simulink model "model_2_type"  (R2022b)
settings: Solver=VariableStepAuto  StartTime=0.0  StopTime=2500  MaxStep=1e-3  RelTol=1e-3
undefined symbols (not defined in the file or in its folder): a0, a1, b0, gamma_1, gamma_2, k0, k_M_1, k_M_2
settings Model: Creator=deniskirbaba  LastModifiedBy=R1303-We2-1-Stud
settings OptimizationCC: ReuseModelBlockBuffer=on

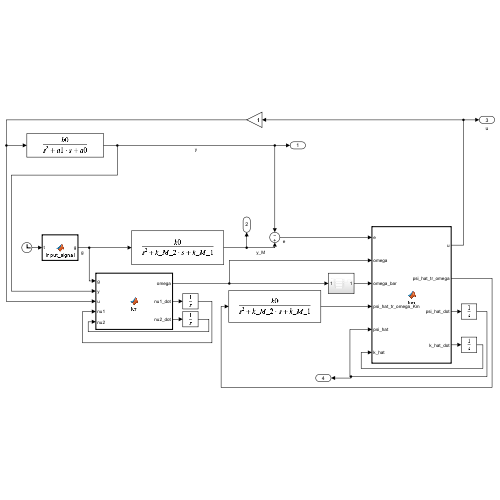
[thumbnail: Simulink's stored preview of the top-level diagram]
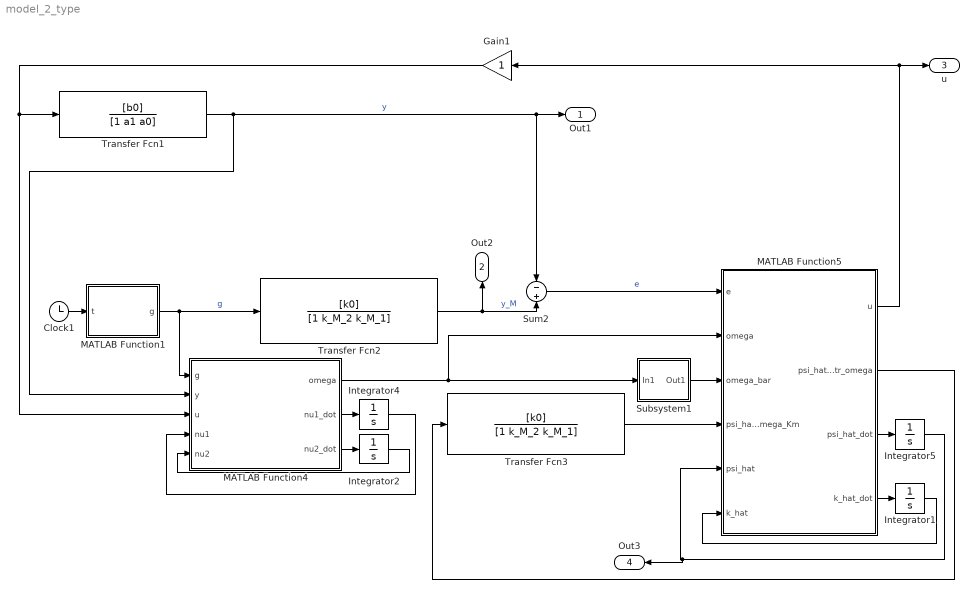
== system model_2_type ==
  Clock1 : Clock
  Gain1 : Gain
  Integrator1 : Integrator
  Integrator2 : Integrator
  Integrator4 : Integrator
  Integrator5 : Integrator  InitialCondition=[0;0;0;0]
  MATLAB Function1 : MATLAB Function  TreatAsAtomicUnit=on
  MATLAB Function4 : MATLAB Function  TreatAsAtomicUnit=on
  MATLAB Function5 : MATLAB Function  TreatAsAtomicUnit=on
  Subsystem1 : Subsystem
  Sum2 : Sum  Inputs=-+
  Transfer Fcn1 : TransferFcn  Numerator=[b0]  Denominator=[1 a1 a0]
  Transfer Fcn2 : TransferFcn  Numerator=[k0]  Denominator=[1 k_M_2 k_M_1]
  Transfer Fcn3 : TransferFcn  Numerator=[k0]  Denominator=[1 k_M_2 k_M_1]
  Out1 : Outport
  Out2 : Outport  Port=2
  u : Outport  Port=3
  Out3 : Outport  Port=4
  wires:
  MATLAB Function4/2(nu1_dot) -> Integrator4/1
  MATLAB Function1/1(g) -> MATLAB Function4/1(g), Transfer Fcn2/1  "g"
  Transfer Fcn2/1 -> Out2/1, Sum2/2  "y_M"
  MATLAB Function5/2(psi_hat_tr_omega) -> Transfer Fcn3/1
  Transfer Fcn3/1 -> MATLAB Function5/4(psi_hat_tr_omega_Km)
  MATLAB Function4/1(omega) -> Subsystem1/1(In1), MATLAB Function5/2(omega)
  Gain1/1 -> MATLAB Function4/3(u), Transfer Fcn1/1
  Clock1/1 -> MATLAB Function1/1(t)
  Subsystem1/1(Out1) -> MATLAB Function5/3(omega_bar)
  Integrator2/1 -> MATLAB Function4/5(nu2)
  Transfer Fcn1/1 -> Out1/1, Sum2/1, MATLAB Function4/2(y)  "y"
  MATLAB Function5/3(psi_hat_dot) -> Integrator5/1
  Integrator4/1 -> MATLAB Function4/4(nu1)
  MATLAB Function4/3(nu2_dot) -> Integrator2/1
  Sum2/1 -> MATLAB Function5/1(e)  "e"
  Integrator5/1 -> Out3/1, MATLAB Function5/5(psi_hat)
  MATLAB Function5/1(u) -> u/1, Gain1/1
  MATLAB Function5/4(k_hat_dot) -> Integrator1/1
  Integrator1/1 -> MATLAB Function5/6(k_hat)

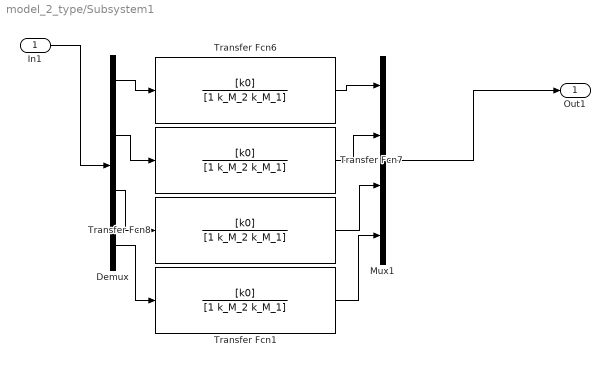
== system model_2_type/Subsystem1 ==
  In1 : Inport
  Demux : Demux
  Mux1 : Mux
  Transfer Fcn{1,6..8} (4 alike) : TransferFcn  Numerator=[k0]  Denominator=[1 k_M_2 k_M_1]
  Out1 : Outport
  wires:
  Transfer Fcn6/1 -> Mux1/1
  Demux/1 -> Transfer Fcn6/1
  Demux/3 -> Transfer Fcn8/1
  Demux/2 -> Transfer Fcn7/1
  Transfer Fcn7/1 -> Mux1/2
  In1/1 -> Demux/1
  Mux1/1 -> Out1/1
  Transfer Fcn8/1 -> Mux1/3
  Demux/4 -> Transfer Fcn1/1
  Transfer Fcn1/1 -> Mux1/4

== matlab function model_2_type/MATLAB Function1 ==
  data: t input; g output
function g = input_signal(t)
    g = sin(t);%7*sign(cos(0.9*t));
end

== matlab function model_2_type/MATLAB Function4 ==
  data: g input; y input; u input; nu1 input; nu2 input; omega output; nu1_dot output; nu2_dot output; k0 parameter
function [omega, nu1_dot, nu2_dot] = fcn(g, y, u, nu1, nu2, k0)
    lambda =-k0;
    
    nu1_dot = lambda*nu1 + u;
    nu2_dot = lambda*nu2 + y;

    omega = [nu1,nu2,y,g]';
end

== matlab function model_2_type/MATLAB Function5 ==
  data: e input; omega input; omega_bar input; psi_hat_tr_omega_Km input; psi_hat input; k_hat input; u output; psi_hat_tr_omega output; psi_hat_dot output; gamma_1 parameter; gamma_2 parameter; k_hat_dot output
function [u, psi_hat_tr_omega, psi_hat_dot, k_hat_dot] = fcn(e, omega, omega_bar, psi_hat_tr_omega_Km, psi_hat, k_hat, gamma_1, gamma_2)
    psi_hat_tr_omega = psi_hat'*omega;
    xi = psi_hat_tr_omega_Km-psi_hat'*omega_bar;
    e_hat = e+k_hat*xi;
    u = psi_hat'*omega;
    psi_hat_dot = gamma_1*omega_bar/(1+omega_bar'*omega_bar)*e_hat;
    k_hat_dot = -gamma_2*xi/(1+omega_bar'*omega_bar)*e_hat;
end
